simulink model "OFDM_Tx_Rx_Loopback"  (R2020a)
settings: Solver=FixedStepDiscrete  StartTime=0.0  StopTime=inf  RelTol=1e-3
InitFcn:
  | % Set parameters
  | fs = 200e3;
  | 
  | % Load all required variables
  | load('read_addr_data');
  | load('read_addr_cp');
  | load('read_addr_pream');
  | load('read_addr_rx');
  | load('pilot');
  | load('LTSfreq');
  | load('STSfreq');
  | load('LTSread');
  | load('STSread');
  | load('bpsk');
  | load('qpsk');
  | load('qam16');
values from neighbouring files (symbols this model uses):
  bpsk = [0 0 1 1 1 1 0 0 1 0 1 0 ... (48 elements, 48x1)]    [bpsk.mat]
  qam16 = [12 5 10 3 14 8 1 10 8 7 2 13 ... (48 elements, 48x1)]    [qam16.mat]
  qpsk = [1 2 1 2 2 2 3 1 1 3 1 0 ... (48 elements, 48x1)]    [qpsk.mat]
  STSfreq = [0 0 0 0 0 0 0 0 1 0 0 0 ... (64 elements, 1x64)]    [STSfreq.mat]
undefined symbols (not defined in the file or in its folder): data3, LTSfreq, LTSread, pilot, read_addr_cp, read_addr_data, read_addr_pream, read_addr_rx, STSread
libraries: hdlsllib x54, simulink x27, dsphdlxfrm x2, dsphdlsigops x1, dsphdlmathfun x1
(part 4 of 4)

== system OFDM_Tx_Rx_Loopback/OFDMRx/Synchronisation/FineTimingSynch/MatchedFilter/Subsystem42 ==
  MatchedIn : Inport
  Add : Sum  OutDataTypeStr=fixdt(1,18,14)
  Add1 : Sum  Inputs=+-  OutDataTypeStr=fixdt(1,18,14)
  Complex to Real-Imag : ComplexToRealImag
  Real-Imag to Complex : RealImagToComplex
  Out1 : Outport
  wires:
  Real-Imag to Complex/1 -> Out1/1
  MatchedIn/1 -> Complex to Real-Imag/1
  Complex to Real-Imag/1 -> Add/1, Add1/2
  Add1/1 -> Real-Imag to Complex/2
  Add/1 -> Real-Imag to Complex/1
  Complex to Real-Imag/2 -> Add/2, Add1/1

== system OFDM_Tx_Rx_Loopback/OFDMRx/Synchronisation/FineTimingSynch/MatchedFilter/Subsystem43 ==
  MatchedIn : Inport
  Add : Sum  OutDataTypeStr=fixdt(1,18,14)
  Add1 : Sum  Inputs=+-  OutDataTypeStr=fixdt(1,18,14)
  Complex to Real-Imag : ComplexToRealImag
  Real-Imag to Complex : RealImagToComplex
  Out1 : Outport
  wires:
  Real-Imag to Complex/1 -> Out1/1
  MatchedIn/1 -> Complex to Real-Imag/1
  Complex to Real-Imag/1 -> Add/1, Add1/2
  Add1/1 -> Real-Imag to Complex/2
  Add/1 -> Real-Imag to Complex/1
  Complex to Real-Imag/2 -> Add/2, Add1/1

== system OFDM_Tx_Rx_Loopback/OFDMRx/Synchronisation/FineTimingSynch/MatchedFilter/Subsystem44 ==
  MatchedIn : Inport
  Add : Sum  OutDataTypeStr=fixdt(1,18,14)
  Add1 : Sum  Inputs=+-  OutDataTypeStr=fixdt(1,18,14)
  Complex to Real-Imag : ComplexToRealImag
  Real-Imag to Complex : RealImagToComplex
  Unary Minus : UnaryMinus
  Out1 : Outport
  wires:
  Real-Imag to Complex/1 -> Out1/1
  MatchedIn/1 -> Complex to Real-Imag/1
  Add1/1 -> Real-Imag to Complex/1
  Complex to Real-Imag/2 -> Add/2, Add1/1
  Complex to Real-Imag/1 -> Add/1, Add1/2
  Add/1 -> Unary Minus/1
  Unary Minus/1 -> Real-Imag to Complex/2

== system OFDM_Tx_Rx_Loopback/OFDMRx/Synchronisation/FineTimingSynch/MatchedFilter/Subsystem45 ==
  MatchedIn : Inport
  Add : Sum  OutDataTypeStr=fixdt(1,18,14)
  Add1 : Sum  Inputs=+-  OutDataTypeStr=fixdt(1,18,14)
  Complex to Real-Imag : ComplexToRealImag
  Real-Imag to Complex : RealImagToComplex
  Unary Minus : UnaryMinus
  Out1 : Outport
  wires:
  Unary Minus/1 -> Real-Imag to Complex/2
  Add/1 -> Unary Minus/1
  Complex to Real-Imag/1 -> Add1/2, Add/1
  Complex to Real-Imag/2 -> Add1/1, Add/2
  Add1/1 -> Real-Imag to Complex/1
  MatchedIn/1 -> Complex to Real-Imag/1
  Real-Imag to Complex/1 -> Out1/1

== system OFDM_Tx_Rx_Loopback/OFDMRx/Synchronisation/FineTimingSynch/MatchedFilter/Subsystem46 ==
  MatchedIn : Inport
  Add : Sum  OutDataTypeStr=fixdt(1,18,14)
  Add1 : Sum  Inputs=+-  OutDataTypeStr=fixdt(1,18,14)
  Complex to Real-Imag : ComplexToRealImag
  Real-Imag to Complex : RealImagToComplex
  Out1 : Outport
  wires:
  Real-Imag to Complex/1 -> Out1/1
  MatchedIn/1 -> Complex to Real-Imag/1
  Complex to Real-Imag/1 -> Add/1, Add1/2
  Add1/1 -> Real-Imag to Complex/2
  Add/1 -> Real-Imag to Complex/1
  Complex to Real-Imag/2 -> Add/2, Add1/1

== system OFDM_Tx_Rx_Loopback/OFDMRx/Synchronisation/FineTimingSynch/MatchedFilter/Subsystem47 ==
  MatchedIn : Inport
  Add : Sum  OutDataTypeStr=fixdt(1,18,14)
  Add1 : Sum  Inputs=+-  OutDataTypeStr=fixdt(1,18,14)
  Complex to Real-Imag : ComplexToRealImag
  Real-Imag to Complex : RealImagToComplex
  Out1 : Outport
  wires:
  Add/1 -> Real-Imag to Complex/2
  Add1/1 -> Real-Imag to Complex/1
  Complex to Real-Imag/2 -> Add/2, Add1/2
  Complex to Real-Imag/1 -> Add/1, Add1/1
  MatchedIn/1 -> Complex to Real-Imag/1
  Real-Imag to Complex/1 -> Out1/1

== system OFDM_Tx_Rx_Loopback/OFDMRx/Synchronisation/FineTimingSynch/MatchedFilter/Subsystem48 ==
  MatchedIn : Inport
  Add : Sum  OutDataTypeStr=fixdt(1,18,14)
  Add1 : Sum  Inputs=+-  OutDataTypeStr=fixdt(1,18,14)
  Complex to Real-Imag : ComplexToRealImag
  Real-Imag to Complex : RealImagToComplex
  Out1 : Outport
  wires:
  Real-Imag to Complex/1 -> Out1/1
  MatchedIn/1 -> Complex to Real-Imag/1
  Complex to Real-Imag/1 -> Add1/1, Add/1
  Complex to Real-Imag/2 -> Add1/2, Add/2
  Add1/1 -> Real-Imag to Complex/1
  Add/1 -> Real-Imag to Complex/2

== system OFDM_Tx_Rx_Loopback/OFDMRx/Synchronisation/FineTimingSynch/MatchedFilter/Subsystem5 ==
  MatchedIn : Inport
  Add : Sum  OutDataTypeStr=fixdt(1,18,14)
  Add1 : Sum  Inputs=+-  OutDataTypeStr=fixdt(1,18,14)
  Complex to Real-Imag : ComplexToRealImag
  Real-Imag to Complex : RealImagToComplex
  Unary Minus : UnaryMinus
  Out1 : Outport
  wires:
  Unary Minus/1 -> Real-Imag to Complex/2
  Add/1 -> Unary Minus/1
  Complex to Real-Imag/1 -> Add1/2, Add/1
  Complex to Real-Imag/2 -> Add1/1, Add/2
  Add1/1 -> Real-Imag to Complex/1
  MatchedIn/1 -> Complex to Real-Imag/1
  Real-Imag to Complex/1 -> Out1/1

== system OFDM_Tx_Rx_Loopback/OFDMRx/Synchronisation/FineTimingSynch/MatchedFilter/Subsystem50 ==
  MatchedIn : Inport
  Add : Sum  OutDataTypeStr=fixdt(1,18,14)
  Add1 : Sum  Inputs=+-  OutDataTypeStr=fixdt(1,18,14)
  Complex to Real-Imag : ComplexToRealImag
  Real-Imag to Complex : RealImagToComplex
  Out1 : Outport
  wires:
  Add/1 -> Real-Imag to Complex/2
  Add1/1 -> Real-Imag to Complex/1
  Complex to Real-Imag/2 -> Add/2, Add1/2
  Complex to Real-Imag/1 -> Add/1, Add1/1
  MatchedIn/1 -> Complex to Real-Imag/1
  Real-Imag to Complex/1 -> Out1/1

== system OFDM_Tx_Rx_Loopback/OFDMRx/Synchronisation/FineTimingSynch/MatchedFilter/Subsystem51 ==
  MatchedIn : Inport
  Add : Sum  OutDataTypeStr=fixdt(1,18,14)
  Add1 : Sum  Inputs=+-  OutDataTypeStr=fixdt(1,18,14)
  Complex to Real-Imag : ComplexToRealImag
  Real-Imag to Complex : RealImagToComplex
  Out1 : Outport
  wires:
  Real-Imag to Complex/1 -> Out1/1
  MatchedIn/1 -> Complex to Real-Imag/1
  Complex to Real-Imag/1 -> Add1/1, Add/1
  Complex to Real-Imag/2 -> Add1/2, Add/2
  Add1/1 -> Real-Imag to Complex/1
  Add/1 -> Real-Imag to Complex/2

== system OFDM_Tx_Rx_Loopback/OFDMRx/Synchronisation/FineTimingSynch/MatchedFilter/Subsystem52 ==
  MatchedIn : Inport
  Add : Sum  OutDataTypeStr=fixdt(1,18,14)
  Add1 : Sum  Inputs=+-  OutDataTypeStr=fixdt(1,18,14)
  Complex to Real-Imag : ComplexToRealImag
  Real-Imag to Complex : RealImagToComplex
  Unary Minus : UnaryMinus
  Out1 : Outport
  wires:
  Unary Minus/1 -> Real-Imag to Complex/1
  Real-Imag to Complex/1 -> Out1/1
  MatchedIn/1 -> Complex to Real-Imag/1
  Complex to Real-Imag/1 -> Add/1, Add1/1
  Add1/1 -> Real-Imag to Complex/2
  Add/1 -> Unary Minus/1
  Complex to Real-Imag/2 -> Add/2, Add1/2

== system OFDM_Tx_Rx_Loopback/OFDMRx/Synchronisation/FineTimingSynch/MatchedFilter/Subsystem53 ==
  MatchedIn : Inport
  Add : Sum  OutDataTypeStr=fixdt(1,18,14)
  Add1 : Sum  Inputs=+-  OutDataTypeStr=fixdt(1,18,14)
  Complex to Real-Imag : ComplexToRealImag
  Real-Imag to Complex : RealImagToComplex
  Out1 : Outport
  wires:
  Add/1 -> Real-Imag to Complex/2
  Add1/1 -> Real-Imag to Complex/1
  Complex to Real-Imag/2 -> Add/2, Add1/2
  Complex to Real-Imag/1 -> Add/1, Add1/1
  MatchedIn/1 -> Complex to Real-Imag/1
  Real-Imag to Complex/1 -> Out1/1

== system OFDM_Tx_Rx_Loopback/OFDMRx/Synchronisation/FineTimingSynch/MatchedFilter/Subsystem54 ==
  MatchedIn : Inport
  Add : Sum  OutDataTypeStr=fixdt(1,18,14)
  Add1 : Sum  Inputs=+-  OutDataTypeStr=fixdt(1,18,14)
  Complex to Real-Imag : ComplexToRealImag
  Real-Imag to Complex : RealImagToComplex
  Out1 : Outport
  wires:
  Real-Imag to Complex/1 -> Out1/1
  MatchedIn/1 -> Complex to Real-Imag/1
  Complex to Real-Imag/1 -> Add/1, Add1/2
  Add1/1 -> Real-Imag to Complex/2
  Add/1 -> Real-Imag to Complex/1
  Complex to Real-Imag/2 -> Add/2, Add1/1

== system OFDM_Tx_Rx_Loopback/OFDMRx/Synchronisation/FineTimingSynch/MatchedFilter/Subsystem55 ==
  MatchedIn : Inport
  Add : Sum  OutDataTypeStr=fixdt(1,18,14)
  Add1 : Sum  Inputs=+-  OutDataTypeStr=fixdt(1,18,14)
  Complex to Real-Imag : ComplexToRealImag
  Real-Imag to Complex : RealImagToComplex
  Out1 : Outport
  wires:
  Add/1 -> Real-Imag to Complex/2
  Add1/1 -> Real-Imag to Complex/1
  Complex to Real-Imag/2 -> Add/2, Add1/2
  Complex to Real-Imag/1 -> Add/1, Add1/1
  MatchedIn/1 -> Complex to Real-Imag/1
  Real-Imag to Complex/1 -> Out1/1

== system OFDM_Tx_Rx_Loopback/OFDMRx/Synchronisation/FineTimingSynch/MatchedFilter/Subsystem56 ==
  MatchedIn : Inport
  Add : Sum  OutDataTypeStr=fixdt(1,18,14)
  Add1 : Sum  Inputs=+-  OutDataTypeStr=fixdt(1,18,14)
  Complex to Real-Imag : ComplexToRealImag
  Real-Imag to Complex : RealImagToComplex
  Unary Minus : UnaryMinus
  Out1 : Outport
  wires:
  Unary Minus/1 -> Real-Imag to Complex/1
  Real-Imag to Complex/1 -> Out1/1
  MatchedIn/1 -> Complex to Real-Imag/1
  Complex to Real-Imag/1 -> Add/1, Add1/1
  Add1/1 -> Real-Imag to Complex/2
  Add/1 -> Unary Minus/1
  Complex to Real-Imag/2 -> Add/2, Add1/2

== system OFDM_Tx_Rx_Loopback/OFDMRx/Synchronisation/FineTimingSynch/MatchedFilter/Subsystem57 ==
  MatchedIn : Inport
  Add : Sum  OutDataTypeStr=fixdt(1,18,14)
  Add1 : Sum  Inputs=+-  OutDataTypeStr=fixdt(1,18,14)
  Complex to Real-Imag : ComplexToRealImag
  Real-Imag to Complex : RealImagToComplex
  Unary Minus : UnaryMinus
  Out1 : Outport
  wires:
  Unary Minus/1 -> Real-Imag to Complex/1
  Real-Imag to Complex/1 -> Out1/1
  MatchedIn/1 -> Complex to Real-Imag/1
  Complex to Real-Imag/1 -> Add/1, Add1/1
  Add1/1 -> Real-Imag to Complex/2
  Add/1 -> Unary Minus/1
  Complex to Real-Imag/2 -> Add/2, Add1/2

== system OFDM_Tx_Rx_Loopback/OFDMRx/Synchronisation/FineTimingSynch/MatchedFilter/Subsystem58 ==
  MatchedIn : Inport
  Add : Sum  OutDataTypeStr=fixdt(1,18,14)
  Add1 : Sum  Inputs=+-  OutDataTypeStr=fixdt(1,18,14)
  Complex to Real-Imag : ComplexToRealImag
  Real-Imag to Complex : RealImagToComplex
  Out1 : Outport
  wires:
  Add/1 -> Real-Imag to Complex/2
  Add1/1 -> Real-Imag to Complex/1
  Complex to Real-Imag/2 -> Add/2, Add1/2
  Complex to Real-Imag/1 -> Add/1, Add1/1
  MatchedIn/1 -> Complex to Real-Imag/1
  Real-Imag to Complex/1 -> Out1/1

== system OFDM_Tx_Rx_Loopback/OFDMRx/Synchronisation/FineTimingSynch/MatchedFilter/Subsystem59 ==
  MatchedIn : Inport
  Add : Sum  OutDataTypeStr=fixdt(1,18,14)
  Add1 : Sum  Inputs=+-  OutDataTypeStr=fixdt(1,18,14)
  Complex to Real-Imag : ComplexToRealImag
  Real-Imag to Complex : RealImagToComplex
  Out1 : Outport
  wires:
  Real-Imag to Complex/1 -> Out1/1
  MatchedIn/1 -> Complex to Real-Imag/1
  Complex to Real-Imag/1 -> Add/1, Add1/2
  Add1/1 -> Real-Imag to Complex/2
  Add/1 -> Real-Imag to Complex/1
  Complex to Real-Imag/2 -> Add/2, Add1/1

== system OFDM_Tx_Rx_Loopback/OFDMRx/Synchronisation/FineTimingSynch/MatchedFilter/Subsystem6 ==
  MatchedIn : Inport
  Add : Sum  OutDataTypeStr=fixdt(1,18,14)
  Add1 : Sum  Inputs=+-  OutDataTypeStr=fixdt(1,18,14)
  Complex to Real-Imag : ComplexToRealImag
  Real-Imag to Complex : RealImagToComplex
  Unary Minus : UnaryMinus
  Out1 : Outport
  wires:
  Real-Imag to Complex/1 -> Out1/1
  MatchedIn/1 -> Complex to Real-Imag/1
  Add1/1 -> Real-Imag to Complex/1
  Complex to Real-Imag/2 -> Add/2, Add1/1
  Complex to Real-Imag/1 -> Add/1, Add1/2
  Add/1 -> Unary Minus/1
  Unary Minus/1 -> Real-Imag to Complex/2

== system OFDM_Tx_Rx_Loopback/OFDMRx/Synchronisation/FineTimingSynch/MatchedFilter/Subsystem60 ==
  MatchedIn : Inport
  Add : Sum  OutDataTypeStr=fixdt(1,18,14)
  Add1 : Sum  Inputs=+-  OutDataTypeStr=fixdt(1,18,14)
  Complex to Real-Imag : ComplexToRealImag
  Real-Imag to Complex : RealImagToComplex
  Out1 : Outport
  wires:
  Complex to Real-Imag/2 -> Add1/1, Add/2
  Add/1 -> Real-Imag to Complex/1
  Add1/1 -> Real-Imag to Complex/2
  Complex to Real-Imag/1 -> Add1/2, Add/1
  MatchedIn/1 -> Complex to Real-Imag/1
  Real-Imag to Complex/1 -> Out1/1

== system OFDM_Tx_Rx_Loopback/OFDMRx/Synchronisation/FineTimingSynch/MatchedFilter/Subsystem61 ==
  MatchedIn : Inport
  Add : Sum  OutDataTypeStr=fixdt(1,18,14)
  Add1 : Sum  Inputs=+-  OutDataTypeStr=fixdt(1,18,14)
  Complex to Real-Imag : ComplexToRealImag
  Real-Imag to Complex : RealImagToComplex
  Out1 : Outport
  wires:
  Add/1 -> Real-Imag to Complex/2
  Add1/1 -> Real-Imag to Complex/1
  Complex to Real-Imag/2 -> Add/2, Add1/2
  Complex to Real-Imag/1 -> Add/1, Add1/1
  MatchedIn/1 -> Complex to Real-Imag/1
  Real-Imag to Complex/1 -> Out1/1

== system OFDM_Tx_Rx_Loopback/OFDMRx/Synchronisation/FineTimingSynch/MatchedFilter/Subsystem62 ==
  MatchedIn : Inport
  Add : Sum  OutDataTypeStr=fixdt(1,18,14)
  Add1 : Sum  Inputs=+-  OutDataTypeStr=fixdt(1,18,14)
  Complex to Real-Imag : ComplexToRealImag
  Real-Imag to Complex : RealImagToComplex
  Unary Minus : UnaryMinus
  Out1 : Outport
  wires:
  Unary Minus/1 -> Real-Imag to Complex/1
  Real-Imag to Complex/1 -> Out1/1
  MatchedIn/1 -> Complex to Real-Imag/1
  Complex to Real-Imag/1 -> Add/1, Add1/1
  Add1/1 -> Real-Imag to Complex/2
  Add/1 -> Unary Minus/1
  Complex to Real-Imag/2 -> Add/2, Add1/2

== system OFDM_Tx_Rx_Loopback/OFDMRx/Synchronisation/FineTimingSynch/MatchedFilter/Subsystem63 ==
  MatchedIn : Inport
  Add : Sum  OutDataTypeStr=fixdt(1,18,14)
  Add1 : Sum  Inputs=+-  OutDataTypeStr=fixdt(1,18,14)
  Complex to Real-Imag : ComplexToRealImag
  Real-Imag to Complex : RealImagToComplex
  Unary Minus : UnaryMinus
  Out1 : Outport
  wires:
  Real-Imag to Complex/1 -> Out1/1
  MatchedIn/1 -> Complex to Real-Imag/1
  Add1/1 -> Real-Imag to Complex/1
  Complex to Real-Imag/2 -> Add/2, Add1/1
  Complex to Real-Imag/1 -> Add/1, Add1/2
  Add/1 -> Unary Minus/1
  Unary Minus/1 -> Real-Imag to Complex/2

== system OFDM_Tx_Rx_Loopback/OFDMRx/Synchronisation/FineTimingSynch/MatchedFilter/Subsystem7 ==
  MatchedIn : Inport
  Add : Sum  OutDataTypeStr=fixdt(1,18,14)
  Add1 : Sum  Inputs=+-  OutDataTypeStr=fixdt(1,18,14)
  Complex to Real-Imag : ComplexToRealImag
  Real-Imag to Complex : RealImagToComplex
  Out1 : Outport
  wires:
  Real-Imag to Complex/1 -> Out1/1
  MatchedIn/1 -> Complex to Real-Imag/1
  Complex to Real-Imag/1 -> Add/1, Add1/2
  Add1/1 -> Real-Imag to Complex/2
  Add/1 -> Real-Imag to Complex/1
  Complex to Real-Imag/2 -> Add/2, Add1/1

== system OFDM_Tx_Rx_Loopback/OFDMRx/Synchronisation/FineTimingSynch/MatchedFilter/Subsystem8 ==
  MatchedIn : Inport
  Add : Sum  OutDataTypeStr=fixdt(1,18,14)
  Add1 : Sum  Inputs=+-  OutDataTypeStr=fixdt(1,18,14)
  Complex to Real-Imag : ComplexToRealImag
  Real-Imag to Complex : RealImagToComplex
  Out1 : Outport
  wires:
  Add/1 -> Real-Imag to Complex/2
  Add1/1 -> Real-Imag to Complex/1
  Complex to Real-Imag/2 -> Add/2, Add1/2
  Complex to Real-Imag/1 -> Add/1, Add1/1
  MatchedIn/1 -> Complex to Real-Imag/1
  Real-Imag to Complex/1 -> Out1/1

== system OFDM_Tx_Rx_Loopback/OFDMRx/Synchronisation/FineTimingSynch/MatchedFilter/Subsystem9 ==
  MatchedIn : Inport
  Add : Sum  OutDataTypeStr=fixdt(1,18,14)
  Add1 : Sum  Inputs=+-  OutDataTypeStr=fixdt(1,18,14)
  Complex to Real-Imag : ComplexToRealImag
  Real-Imag to Complex : RealImagToComplex
  Out1 : Outport
  wires:
  Real-Imag to Complex/1 -> Out1/1
  MatchedIn/1 -> Complex to Real-Imag/1
  Complex to Real-Imag/1 -> Add/1, Add1/2
  Add1/1 -> Real-Imag to Complex/2
  Add/1 -> Real-Imag to Complex/1
  Complex to Real-Imag/2 -> Add/2, Add1/1

== system OFDM_Tx_Rx_Loopback/OFDMRx/Synchronisation/CoarseTiming/CoarseTimeStrobeGen/LocalSearchCounter/RsingEdge ==
  In1 : Inport
  Delay : Delay  DelayLength=1
  Relational Operator : RelationalOperator  Operator=>  OutDataTypeStr=boolean  RndMeth=Nearest
  Out1 : Outport  VectorParamsAs1DForOutWhenUnconnected=off
  wires:
  Relational Operator/1 -> Out1/1
  Delay/1 -> Relational Operator/2
  In1/1 -> Delay/1, Relational Operator/1

== matlab function OFDM_Tx_Rx_Loopback/OFDMTx/DataGenerator/Data Multiplexer ==
  data: symbols input; dataready input; data output; pilots input; pval input; sts input; stsval input; lts input; ltsval input
function data  = dataMux(symbols,dataready,pilots,pval,sts,stsval,lts,ltsval)
% Data multiplexer 
if (pval == true)
    data = pilots; 
elseif (stsval == true)
    data = sts; 
elseif (ltsval == true)
    data = lts; 
elseif (dataready == true) 
    data = symbols;
else 
    data = fi(complex(0),1,16,14);
end

== matlab function OFDM_Tx_Rx_Loopback/OFDMTx/SCMapper/Mux2 ==
  data: preamb input; preambVal input; dataOut output; data input; dataVal input
function dataOut = mux(preamb,preambVal,data,dataVal)

if (preambVal == true)
    dataOut = preamb; 
elseif (dataVal == true)
    dataOut = data; 
else 
    dataOut = fi(complex(0),1,16,14);
end

== matlab function OFDM_Tx_Rx_Loopback/OFDMTx/CPAdd/Mux2 ==
  data: sts input; stsval input; lts input; ltsval input; dataOut output; data input; dataval input
function dataOut = mux(sts,stsval,lts,ltsval,data,dataval)

if (stsval == true)
    dataOut = sts; 
elseif (ltsval == true)
    dataOut = lts; 
elseif (dataval == true) 
    dataOut = data; 
else 
    dataOut = fi(complex(0),1,16,14);
end
